simulink model "hydra_tail"  (R2014b)
settings: configuration reference "HardwareConfigLeg" (kept outside this file)
undefined symbols (not defined in the file or in its folder): gcbh, LCD_Status, NXTFcns, R, rmidispblock, Speak, W
libraries: legoev3lib x13, ControllersFcns x5, simulink_extras x4, simulink x3
PreSaveFcn:
  | % Creates new data dictionary based on template.
  | 
  | projRoot = ETRoboconUtilities.getCheckoutRoot;
  | dictName = [bdroot 'Data.sldd'];
  | 
  | source = fullfile(projRoot,'templates','RobotTemplateData.sldd');
  | dest = fullfile(projRoot,'data_dictionaries',dictName);
  | 
  | if ~exist(dest) && ~isequal(bdroot,'RobotTemplate')
  |   copyfile(source,dest);
  |   disp(['Created new dictionary ' dictName ' in the data_dictionaries folder.']);
  |   set_param(bdroot,'DataDictionary', dictName);
  | end
Description:
  | ET Robocon 2014 robot template model.
  | 
  | Author:  Sebastian Castro
settings Model: DataDictionary=hydra_tailData.sldd  ExtModeTrigDuration=2  Creator=mbiesiad  LastModifiedBy=pkaniara

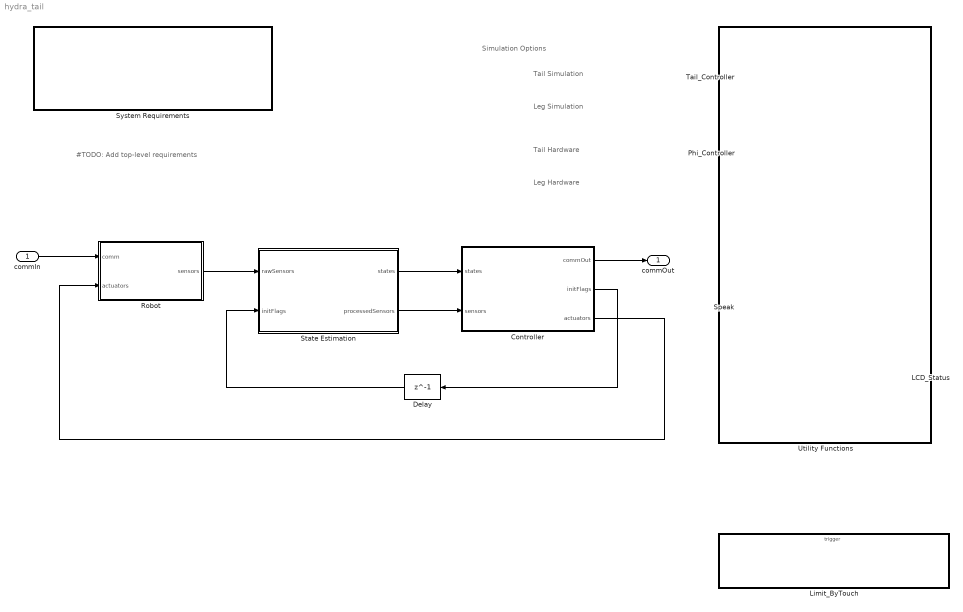
== system hydra_tail ==
  note: #TODO:
      | Add top-level requirements
  note: Simulation Options
  note: Tail Simulation
  note: Tail Hardware
  note: Leg Hardware
  note: Leg Simulation
  commIn : Inport
  Controller : Stateflow chart  TreatAsAtomicUnit=on
  Delay : Delay  DelayLength=1
      settings: AttributesFormatString=Removes algebraic loop
  LCD_Status : Subsystem  AncestorBlock=NXTFcns/LCD_Status  TreatAsAtomicUnit=on
  Limit_ByTouch : Subsystem  TreatAsAtomicUnit=on
  Phi_Controller : ControllersFcns/Phi_Controller
  Robot : Subsystem  Variant=on  VariantControl=Variant1
  Speak : Subsystem  AncestorBlock=NXTFcns/Speak  TreatAsAtomicUnit=on
  State Estimation : Subsystem
  System Requirements : Subsystem  LoadFcn=rmidispblock('load',gcbh)  mask(System Requirements){id=SystemReq, title=System Requirements}
      mask prompts: title "Block Title"
      mask help: Lists the requirements for the current model.
      mask init:
      | id = 'SystemReq';
      | [w,h] = rmidispblock('display',gcbh);
      settings: CopyFcn=rmidispblock('create',gcbh)  DeleteFcn=rmidispblock('delete',gcbh)  ModelCloseFcn=rmidispblock('close',gcbh)  PreSaveFcn=rmidispblock('close',gcbh)  PostSaveFcn=rmidispblock('open',gcbh)  OpenFcn=rmidispblock('open',gcbh)  MoveFcn=rmidispblock('move',gcbh)
      mask Help: helpview(fullfile(docroot,'toolbox','slvnv','slvnv.map'),'systemrequirements')
      mask Display:
      | text(326/2,113-4,rmidispblock('title',gcbh),'horizontalAlignment','center','verticalAlignment','top')
      | text(w/2,h/2,'<No Requirements in System>','horizontalAlignment','center','verticalAlignment','top')
  Tail_Controller : ControllersFcns/Tail_Controller
  Utility Functions : Subsystem
  commOut : Outport
  wires:
  State Estimation/2(processedSensors) -> Controller/2(sensors)
  Robot/1(sensors) -> State Estimation/1(rawSensors)
  Controller/2(initFlags) -> Delay/1
  State Estimation/1(states) -> Controller/1(states)
  Delay/1 -> State Estimation/2(initFlags)
  Controller/3(actuators) -> Robot/2(actuators)
  Controller/1(commOut) -> commOut/1
  commIn/1 -> Robot/1(comm)

== system hydra_tail/Controller/Speak ==
  f : TriggerPort  TriggerType=function-call
      settings: CopyFcn=Stateflow.SLINSF.SimulinkMan.removeBlockPreDeleteFcn  PreDeleteFcn=Stateflow.SLINSF.SimulinkMan.unsafePredeleteFcn
  Constant : Constant  Value=50
  Speaker1 : legoev3lib/Speaker  sinputMode=Volume only  sspeakerFreq=100  sspeakerVolume=50  sspeakerDuration=100
  wires:
  Constant/1 -> Speaker1/1

== system hydra_tail/LCD_Status ==
  StatusLCD : TriggerPort  TriggerType=function-call  IsSimulinkFunction=on  FunctionName=StatusLCD
  Display : legoev3lib/Display  slcdLine=1  slcdFormat=Decimal
  state : ArgIn  OutDataTypeStr=uint16  ArgumentName=state
  wires:
  state/1 -> Display/1

== system hydra_tail/Limit_ByTouch ==
  LimitByTouch : TriggerPort  TriggerType=function-call  IsSimulinkFunction=on  FunctionName=LimitByTouch
  Chart : Stateflow chart  TreatAsAtomicUnit=on
  Compare To Zero : simulink/Logic and Bit Operations/Compare To Zero  relop=>=  OutDataTypeStr=boolean
  Delay : Delay  DelayLength=1
  TouchInput : ArgIn  DisableCoverage=on  ArgumentName=TouchInput
  cmd : ArgOut  DisableCoverage=on  ArgumentName=cmd
  wires:
  TouchInput/1 -> Chart/1(touchInput)
  Chart/1(motorCommand) -> Delay/1, cmd/1
  Delay/1 -> Compare To Zero/1
  Compare To Zero/1 -> Chart/2(direction)

== system hydra_tail/Robot ==
  comm : Inport
  actuators : Inport  Port=2
  EV3 - Legs : Subsystem  VariantControl=HardwareVar2
  EV3 - Tail : Subsystem  VariantControl=HardwareVar1
  Simulation - Legs : Subsystem  VariantControl=SimulationVar2
  Simulation - Tail : Subsystem  VariantControl=SimulationVar1
  sensors : Outport

== system hydra_tail/Speak ==
  Speak : TriggerPort  TriggerType=function-call  IsSimulinkFunction=on  FunctionName=Speak
  Constant : Constant  Value=50
  Speaker1 : legoev3lib/Speaker  sinputMode=Volume only  sspeakerFreq=100  sspeakerVolume=50  sspeakerDuration=100
  wires:
  Constant/1 -> Speaker1/1

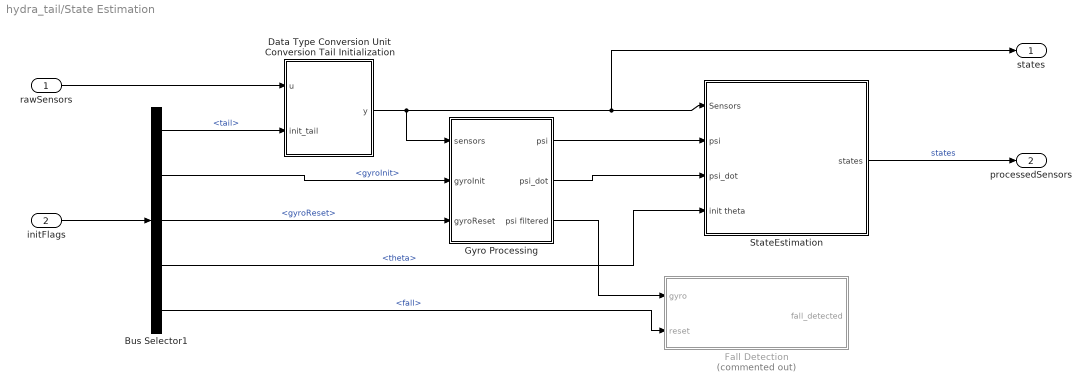
== system hydra_tail/State Estimation ==
  rawSensors : Inport
  initFlags : Inport  Port=2
  Bus Selector1 : BusSelector  OutputSignals=tail,gyroInit,gyroReset,theta,fall
  Data Type Conversion Unit Conversion Tail Initialization : Subsystem
  Fall Detection : Subsystem  Commented=on
  Gyro Processing : Subsystem
  StateEstimation : Subsystem
  states : Outport
  processedSensors : Outport  Port=2
  wires:
  Data Type Conversion Unit Conversion Tail Initialization/1(y) -> Gyro Processing/1(sensors), states/1, StateEstimation/1(Sensors)
  Bus Selector1/3 -> Gyro Processing/3(gyroReset)  "<gyroReset>"
  Bus Selector1/4 -> StateEstimation/4(init theta)  "<theta>"
  Bus Selector1/1 -> Data Type Conversion Unit Conversion Tail Initialization/2(init_tail)  "<tail>"
  Bus Selector1/2 -> Gyro Processing/2(gyroInit)  "<gyroInit>"
  initFlags/1 -> Bus Selector1/1
  StateEstimation/1(states) -> processedSensors/1  "states"
  rawSensors/1 -> Data Type Conversion Unit Conversion Tail Initialization/1(u)
  Gyro Processing/1(psi) -> StateEstimation/2(psi)
  Gyro Processing/2(psi_dot) -> StateEstimation/3(psi_dot)
  Gyro Processing/3(psi filtered) -> Fall Detection/1(gyro)
  Bus Selector1/5 -> Fall Detection/2(reset)  "<fall>"

== system hydra_tail/System Requirements ==
  Subsystem : Subsystem  mask{label=0, index=1}
      mask init:
      | label = rmidispblock('label',index);
      settings: OpenFcn=rmidispblock('openReq',gcbh);
      mask Display: text(0,0,label,'horizontalAlignment','left','verticalAlignment','bottom')

== system hydra_tail/Utility Functions ==

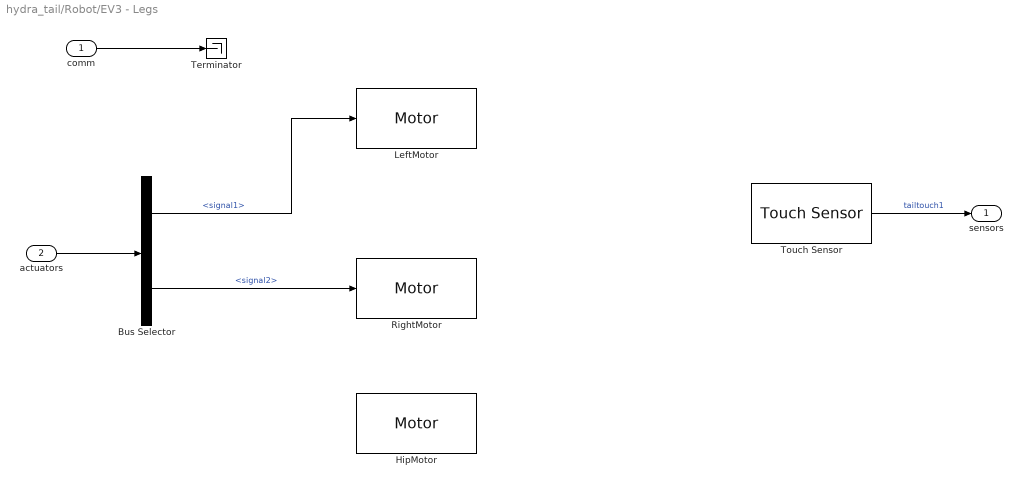
== system hydra_tail/Robot/EV3 - Legs ==
  comm : Inport
  actuators : Inport  Port=2
  Bus Selector : BusSelector  OutputSignals=signal1,signal2
  HipMotor : legoev3lib/Motor  sportNumber=C  sstopAction=Brake
  LeftMotor : legoev3lib/Motor  sportNumber=A  sstopAction=Brake
  RightMotor : legoev3lib/Motor  sportNumber=B  sstopAction=Brake
  Terminator : Terminator
  Touch Sensor : legoev3lib/Touch Sensor  portNumber=1  sampleTime=0.1
  sensors : Outport
  wires:
  comm/1 -> Terminator/1
  Touch Sensor/1 -> sensors/1  "tailtouch1"
  Bus Selector/1 -> LeftMotor/1  "<signal1>"
  actuators/1 -> Bus Selector/1
  Bus Selector/2 -> RightMotor/1  "<signal2>"

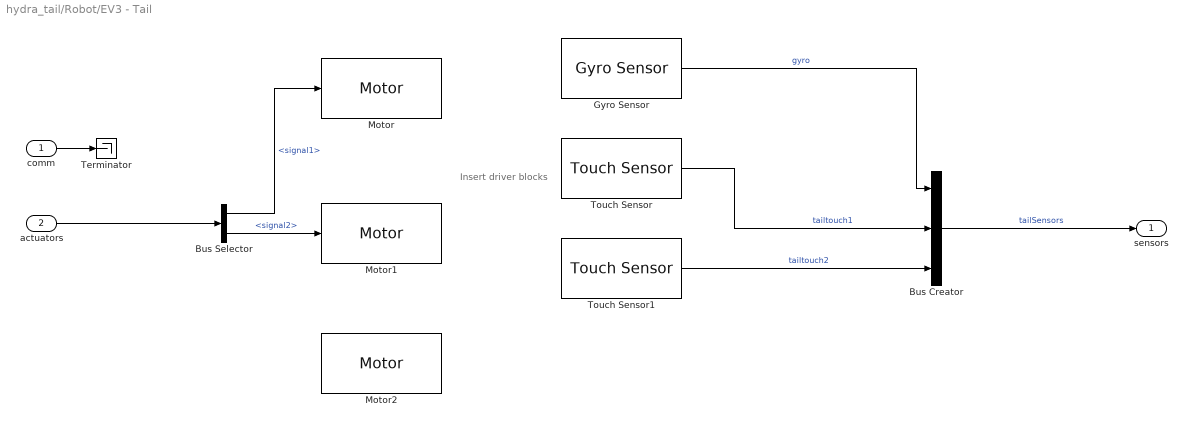
== system hydra_tail/Robot/EV3 - Tail ==
  note: Insert driver blocks
  comm : Inport
  actuators : Inport  Port=2
  Bus Creator : BusCreator  Inputs=3
  Bus Selector : BusSelector  OutputSignals=signal1,signal2
  Gyro Sensor : legoev3lib/Gyro Sensor  portNumber=1  sampleTime=0.1
  Motor : legoev3lib/Motor  sportNumber=A  sstopAction=Brake
  Motor1 : legoev3lib/Motor  sportNumber=B  sstopAction=Brake
  Motor2 : legoev3lib/Motor  sportNumber=C  sstopAction=Brake
  Terminator : Terminator
  Touch Sensor : legoev3lib/Touch Sensor  portNumber=1  sampleTime=0.1
  Touch Sensor1 : legoev3lib/Touch Sensor  portNumber=1  sampleTime=0.1
  sensors : Outport
  wires:
  Bus Creator/1 -> sensors/1  "tailSensors"
  actuators/1 -> Bus Selector/1
  comm/1 -> Terminator/1
  Gyro Sensor/1 -> Bus Creator/1  "gyro"
  Touch Sensor/1 -> Bus Creator/2  "tailtouch1"
  Touch Sensor1/1 -> Bus Creator/3  "tailtouch2"
  Bus Selector/1 -> Motor/1  "<signal1>"
  Bus Selector/2 -> Motor1/1  "<signal2>"

== system hydra_tail/Robot/Simulation - Legs ==
  note: Insert physical model.
      | Talk to the simulation team!
  comm : Inport
  actuators : Inport  Port=2
  Ground : Ground
  Terminator : Terminator
  Terminator1 : Terminator
  sensors : Outport
  wires:
  comm/1 -> Terminator/1
  actuators/1 -> Terminator1/1
  Ground/1 -> sensors/1

== system hydra_tail/Robot/Simulation - Tail ==
  note: Insert physical model.
      | Talk to the simulation team!
  comm : Inport
  actuators : Inport  Port=2
  Ground : Ground
  Terminator : Terminator
  Terminator1 : Terminator
  sensors : Outport
  wires:
  Ground/1 -> sensors/1
  actuators/1 -> Terminator1/1
  comm/1 -> Terminator/1

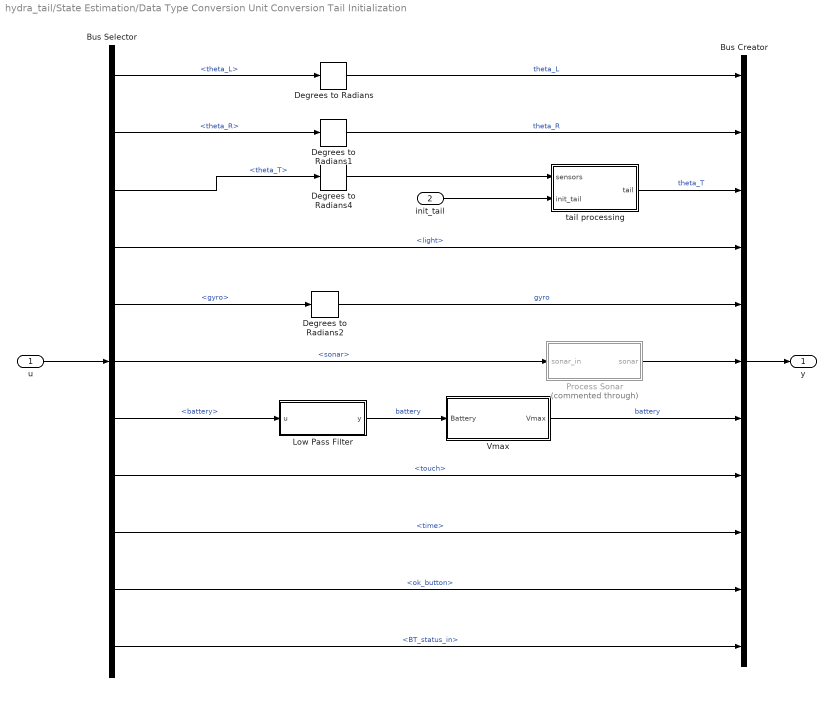
== system hydra_tail/State Estimation/Data Type Conversion Unit Conversion Tail Initialization ==
  u : Inport
  init_tail : Inport  Port=2
  Bus Creator : BusCreator  Inputs=11  OutDataTypeStr=Bus: Sensors_Bus
  Bus Selector : BusSelector  OutputSignals=theta_L,theta_R,theta_T,light,gyro,sonar,battery,touch,time,ok_button,BT_status_in
  Degrees to Radians{,1..2,4} (4 alike) : simulink_extras/Transformations/Degrees to Radians
  Low Pass Filter : Subsystem
  Process Sonar : Subsystem  Commented=through
  Vmax : Subsystem
  tail processing : Subsystem
  y : Outport
  wires:
  Bus Selector/11 -> Bus Creator/11  "<BT_status_in>"
  Process Sonar/1(sonar) -> Bus Creator/6
  Bus Selector/6 -> Process Sonar/1(sonar_in)  "<sonar>"
  Bus Selector/10 -> Bus Creator/10  "<ok_button>"
  init_tail/1 -> tail processing/2(init_tail)
  Bus Selector/9 -> Bus Creator/9  "<time>"
  Bus Selector/8 -> Bus Creator/8  "<touch>"
  tail processing/1(tail) -> Bus Creator/3  "theta_T"
  Degrees to Radians4/1 -> tail processing/1(sensors)
  Vmax/1(Vmax) -> Bus Creator/7  "battery"
  Degrees to Radians2/1 -> Bus Creator/5  "gyro"
  Bus Selector/3 -> Degrees to Radians4/1  "<theta_T>"
  Bus Selector/7 -> Low Pass Filter/1(u)  "<battery>"
  Bus Selector/5 -> Degrees to Radians2/1  "<gyro>"
  Bus Selector/4 -> Bus Creator/4  "<light>"
  Bus Creator/1 -> y/1
  u/1 -> Bus Selector/1
  Degrees to Radians/1 -> Bus Creator/1  "theta_L"
  Bus Selector/2 -> Degrees to Radians1/1  "<theta_R>"
  Bus Selector/1 -> Degrees to Radians/1  "<theta_L>"
  Low Pass Filter/1(y) -> Vmax/1(Battery)  "battery"
  Degrees to Radians1/1 -> Bus Creator/2  "theta_R"

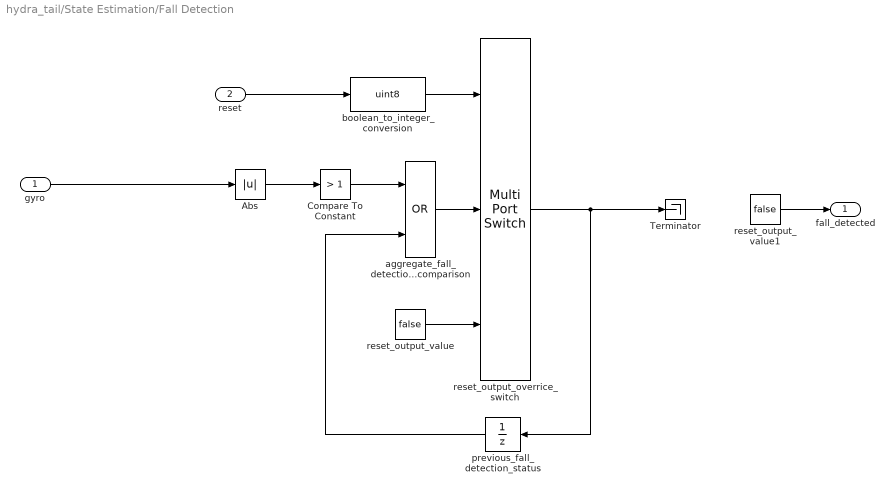
== system hydra_tail/State Estimation/Fall Detection ==
  gyro : Inport
      settings: AttributesFormatString=Output data type: %<OutDataTypeStr>
  reset : Inport  Port=2  OutDataTypeStr=boolean
      settings: AttributesFormatString=Output data type: %<OutDataTypeStr>
  Abs : Abs
  Compare To Constant : simulink/Logic and Bit Operations/Compare To Constant  relop=>  const=1  OutDataTypeStr=boolean
  Terminator : Terminator
  aggregate_fall_detection_comparison : Logic  Operator=OR  OutDataTypeStr=boolean
  boolean_to_integer_conversion : DataTypeConversion  OutDataTypeStr=uint8
      settings: AttributesFormatString=Output data type: %<OutDataTypeStr>
  previous_fall_detection_status : UnitDelay  SampleTime=-1
  reset_output_overrice_switch : MultiPortSwitch  DataPortOrder=Zero-based contiguous  Inputs=2  zeroidx=on  InputSameDT=on
  reset_output_value : Constant  Value=false
  reset_output_value1 : Constant  Value=false  OutDataTypeStr=boolean
  fall_detected : Outport
  wires:
  reset_output_overrice_switch/1 -> Terminator/1, previous_fall_detection_status/1
  reset_output_value/1 -> reset_output_overrice_switch/3
  aggregate_fall_detection_comparison/1 -> reset_output_overrice_switch/2
  boolean_to_integer_conversion/1 -> reset_output_overrice_switch/1
  reset/1 -> boolean_to_integer_conversion/1
  previous_fall_detection_status/1 -> aggregate_fall_detection_comparison/2
  Abs/1 -> Compare To Constant/1
  gyro/1 -> Abs/1
  Compare To Constant/1 -> aggregate_fall_detection_comparison/1
  reset_output_value1/1 -> fall_detected/1

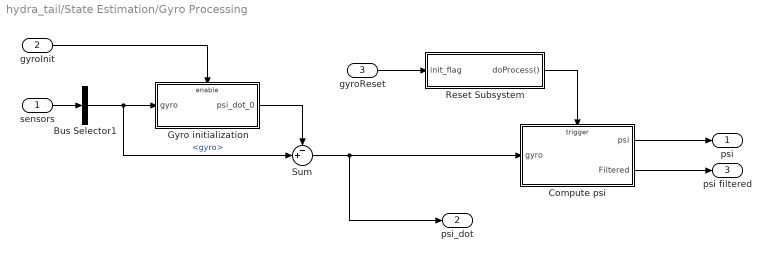
== system hydra_tail/State Estimation/Gyro Processing ==
  sensors : Inport
  gyroInit : Inport  Port=2
  gyroReset : Inport  Port=3
  Bus Selector1 : BusSelector  OutputSignals=gyro
  Compute psi : Subsystem
  Gyro initialization : Subsystem  TreatAsAtomicUnit=on
  Reset Subsystem : Stateflow chart  TreatAsAtomicUnit=on
  Sum : Sum  Inputs=-+|
  psi : Outport
  psi_dot : Outport  Port=2
  psi filtered : Outport  Port=3
  wires:
  Compute psi/2(Filtered) -> psi filtered/1
  Reset Subsystem/1(doProcess()) -> Compute psi/Trigger
  gyroReset/1 -> Reset Subsystem/1(init_flag)
  Bus Selector1/1 -> Sum/2, Gyro initialization/1(gyro)  "<gyro>"
  Gyro initialization/1(psi_dot_0) -> Sum/1
  Sum/1 -> psi_dot/1, Compute psi/1(gyro)
  Compute psi/1(psi) -> psi/1
  sensors/1 -> Bus Selector1/1
  gyroInit/1 -> Gyro initialization/Enable

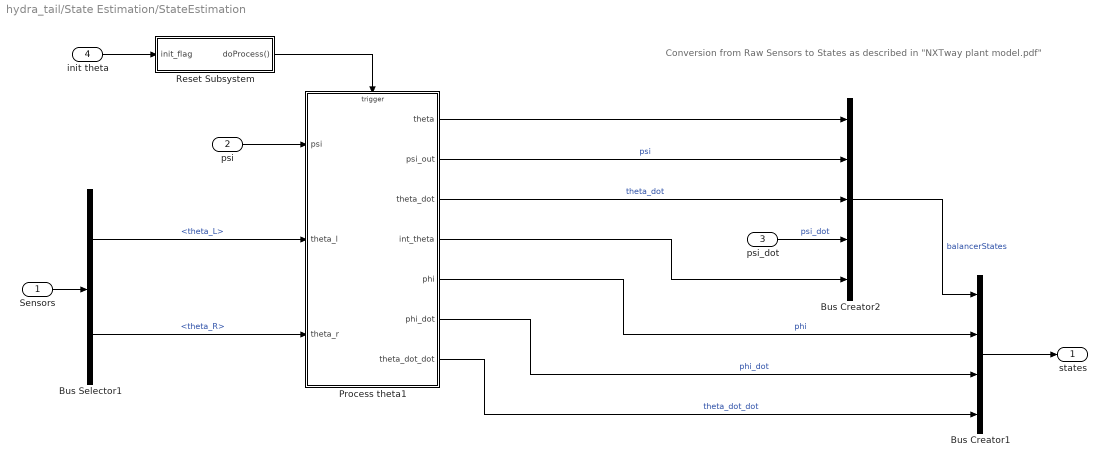
== system hydra_tail/State Estimation/StateEstimation ==
  note: Conversion from Raw Sensors to States as described in "NXTway plant model.pdf"
  Sensors : Inport
  psi : Inport  Port=2
  psi_dot : Inport  Port=3
  init theta : Inport  Port=4
  Bus Creator1 : BusCreator  OutDataTypeStr=Bus: States_Bus
  Bus Creator2 : BusCreator  Inputs=5  OutDataTypeStr=Bus: Balancer_States_Bus
  Bus Selector1 : BusSelector  OutputSignals=theta_L,theta_R
  Process theta1 : Subsystem
  Reset Subsystem : Stateflow chart  TreatAsAtomicUnit=on
  states : Outport  OutputWhenDisabled=reset  InitialOutput=0
  wires:
  Process theta1/2(psi_out) -> Bus Creator2/2  "psi"
  Reset Subsystem/1(doProcess()) -> Process theta1/Trigger
  Bus Selector1/2 -> Process theta1/3(theta_r)  "<theta_R>"
  Bus Selector1/1 -> Process theta1/2(theta_l)  "<theta_L>"
  init theta/1 -> Reset Subsystem/1(init_flag)
  Process theta1/1(theta) -> Bus Creator2/1
  Process theta1/3(theta_dot) -> Bus Creator2/3  "theta_dot"
  Process theta1/4(int_theta) -> Bus Creator2/5
  psi_dot/1 -> Bus Creator2/4  "psi_dot"
  Process theta1/6(phi_dot) -> Bus Creator1/3  "phi_dot"
  Bus Creator2/1 -> Bus Creator1/1  "balancerStates"
  Process theta1/5(phi) -> Bus Creator1/2  "phi"
  Sensors/1 -> Bus Selector1/1
  psi/1 -> Process theta1/1(psi)
  Bus Creator1/1 -> states/1
  Process theta1/7(theta_dot_dot) -> Bus Creator1/4  "theta_dot_dot"

== system hydra_tail/System Requirements/Subsystem ==

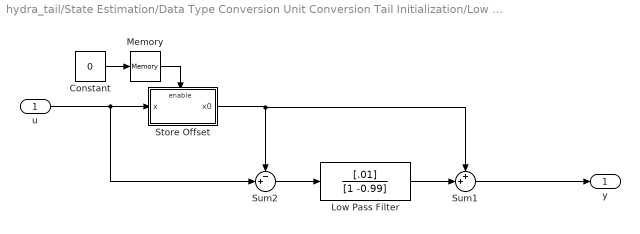
== system hydra_tail/State Estimation/Data Type Conversion Unit Conversion Tail Initialization/Low Pass Filter ==
  u : Inport
  Constant : Constant  Value=0  OutDataTypeStr=boolean
  Low Pass Filter : DiscreteFilter  Numerator=[.01]  Denominator=[1 -0.99]
  Memory : Memory  X0=1  InheritSampleTime=on
  Store Offset : Subsystem  TreatAsAtomicUnit=on
  Sum1 : Sum  Inputs=++|
  Sum2 : Sum  Inputs=-+|
  y : Outport
  wires:
  Store Offset/1(x0) -> Sum1/1, Sum2/1
  u/1 -> Store Offset/1(x), Sum2/2
  Constant/1 -> Memory/1
  Memory/1 -> Store Offset/Enable
  Sum2/1 -> Low Pass Filter/1
  Sum1/1 -> y/1
  Low Pass Filter/1 -> Sum1/2

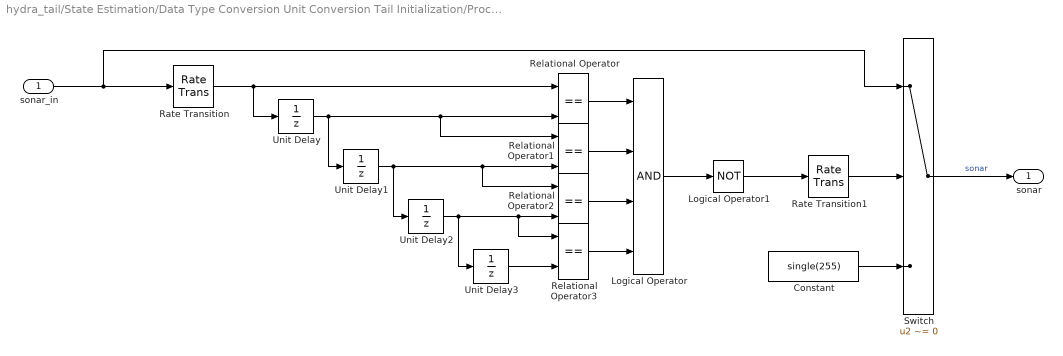
== system hydra_tail/State Estimation/Data Type Conversion Unit Conversion Tail Initialization/Process Sonar ==
  sonar_in : Inport
  Constant : Constant  Value=single(255)
  Logical Operator : Logic  Inputs=4  AllPortsSameDT=off  OutDataTypeStr=boolean
  Logical Operator1 : Logic  Operator=NOT  AllPortsSameDT=off  OutDataTypeStr=boolean
  Rate Transition : RateTransition  OutPortSampleTime=0.02
  Rate Transition1 : RateTransition  OutPortSampleTime=0.004
  Relational Operator{,1..3} (4 alike) : RelationalOperator  Operator===  OutDataTypeStr=boolean
  Switch : Switch  Criteria=u2 ~= 0
  Unit Delay{,1..3} (4 alike) : UnitDelay  SampleTime=-1
  sonar : Outport
  wires:
  Switch/1 -> sonar/1  "sonar"
  Constant/1 -> Switch/3
  Rate Transition1/1 -> Switch/2
  Logical Operator1/1 -> Rate Transition1/1
  Logical Operator/1 -> Logical Operator1/1
  Relational Operator2/1 -> Logical Operator/3
  Relational Operator1/1 -> Logical Operator/2
  Relational Operator3/1 -> Logical Operator/4
  Relational Operator/1 -> Logical Operator/1
  Unit Delay3/1 -> Relational Operator3/2
  Unit Delay2/1 -> Unit Delay3/1, Relational Operator2/2, Relational Operator3/1
  Unit Delay1/1 -> Unit Delay2/1, Relational Operator1/2, Relational Operator2/1
  Unit Delay/1 -> Unit Delay1/1, Relational Operator/2, Relational Operator1/1
  Rate Transition/1 -> Unit Delay/1, Relational Operator/1
  sonar_in/1 -> Rate Transition/1, Switch/1

== system hydra_tail/State Estimation/Data Type Conversion Unit Conversion Tail Initialization/Vmax ==
  Battery : Inport
  Constant : Constant  Value=0.625  OutDataTypeStr=single
  Gain1 : Gain  Gain=0.001089
  Sum : Sum  Inputs=|+-
  Vmax : Outport
  wires:
  Battery/1 -> Gain1/1
  Gain1/1 -> Sum/1
  Constant/1 -> Sum/2
  Sum/1 -> Vmax/1

== system hydra_tail/State Estimation/Data Type Conversion Unit Conversion Tail Initialization/tail processing ==
  sensors : Inport
  init_tail : Inport  Port=2
  Sum : Sum  Inputs=-+|
  tail initialization : Subsystem  TreatAsAtomicUnit=on
  tail : Outport  OutputWhenDisabled=reset  InitialOutput=0
  wires:
  Sum/1 -> tail/1  "theta_T"
  sensors/1 -> Sum/2, tail initialization/1(tail)
  tail initialization/1(tail_0) -> Sum/1
  init_tail/1 -> tail initialization/Trigger

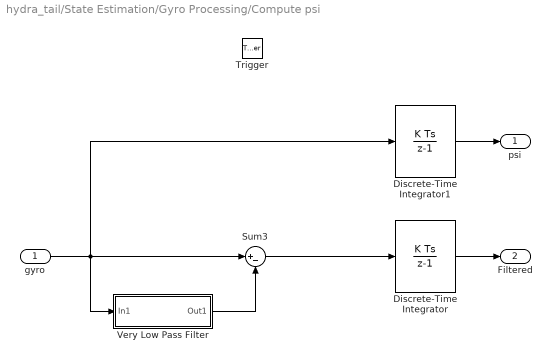
== system hydra_tail/State Estimation/Gyro Processing/Compute psi ==
  gyro : Inport
  Trigger : TriggerPort  TriggerType=function-call  StatesWhenEnabling=reset  PortDimensions=1
  Discrete-Time Integrator : DiscreteIntegrator  SampleTime=-1
  Discrete-Time Integrator1 : DiscreteIntegrator  SampleTime=-1
  Sum3 : Sum  Inputs=|+-
  Very Low Pass Filter : Subsystem
  psi : Outport  InitialOutput=0
  Filtered : Outport  Port=2  InitialOutput=0
  wires:
  Discrete-Time Integrator/1 -> Filtered/1
  Discrete-Time Integrator1/1 -> psi/1
  Sum3/1 -> Discrete-Time Integrator/1
  Very Low Pass Filter/1(Out1) -> Sum3/2
  gyro/1 -> Very Low Pass Filter/1(In1), Sum3/1, Discrete-Time Integrator1/1

== system hydra_tail/State Estimation/Gyro Processing/Gyro initialization ==
  gyro : Inport
  Enable : EnablePort  StatesWhenEnabling=reset
  Low Pass Filter : DiscreteFilter  Numerator=[.01]  Denominator=[1 -0.99]
  psi_dot_0 : Outport  InitialOutput=0
  wires:
  Low Pass Filter/1 -> psi_dot_0/1
  gyro/1 -> Low Pass Filter/1

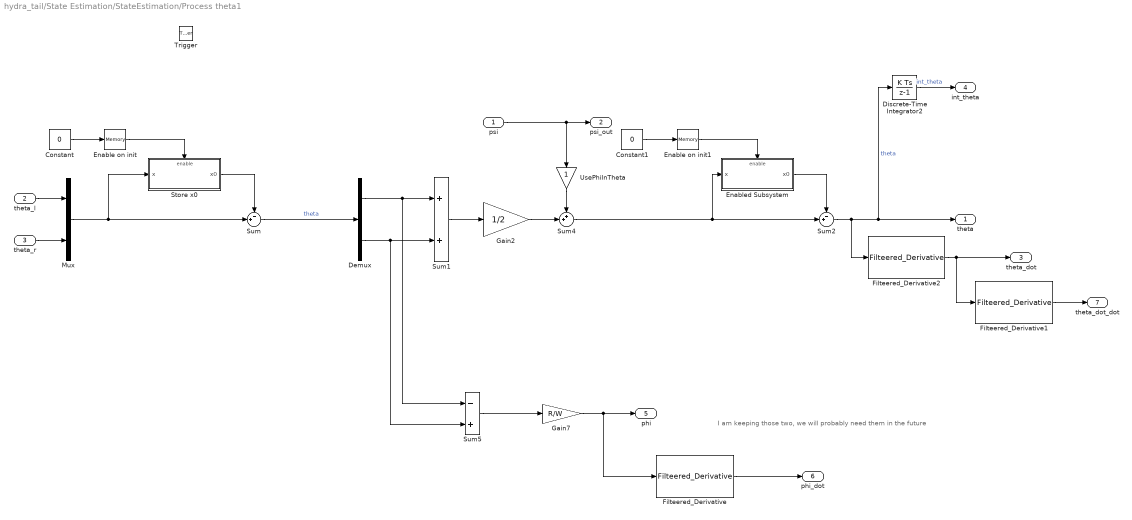
== system hydra_tail/State Estimation/StateEstimation/Process theta1 ==
  note: I am keeping those two, we will probably need them in the future
  psi : Inport
  theta_l : Inport  Port=2
  theta_r : Inport  Port=3
  Trigger : TriggerPort  TriggerType=function-call  StatesWhenEnabling=reset  PortDimensions=1
  Constant : Constant  Value=0  OutDataTypeStr=boolean
  Constant1 : Constant  Value=0  OutDataTypeStr=boolean
  Demux : Demux  Outputs=2
  Discrete-Time Integrator2 : DiscreteIntegrator  SampleTime=-1
  Enable on init : Memory  X0=1  InheritSampleTime=on
  Enable on init1 : Memory  X0=1  InheritSampleTime=on
  Enabled Subsystem : Subsystem  TreatAsAtomicUnit=on
  Filteered_Derivative : ControllersFcns/Filteered_Derivative
  Filteered_Derivative1 : ControllersFcns/Filteered_Derivative
  Filteered_Derivative2 : ControllersFcns/Filteered_Derivative
  Gain2 : Gain  Gain=1/2
  Gain7 : Gain  Gain=R/W
  Mux : Mux  Inputs=2
  Store x0 : Subsystem  TreatAsAtomicUnit=on
  Sum : Sum  Inputs=-+|
  Sum1 : Sum
  Sum2 : Sum  Inputs=-+|
  Sum4 : Sum  Inputs=++|
  Sum5 : Sum  Inputs=-+
  UsePhiInTheta : Gain
  theta : Outport  InitialOutput=0
  psi_out : Outport  Port=2  InitialOutput=0
  theta_dot : Outport  Port=3  OutputWhenDisabled=reset  InitialOutput=0
  int_theta : Outport  Port=4  InitialOutput=0
  phi : Outport  Port=5  OutputWhenDisabled=reset  InitialOutput=0
  phi_dot : Outport  Port=6  OutputWhenDisabled=reset  InitialOutput=0
  theta_dot_dot : Outport  Port=7  OutputWhenDisabled=reset  InitialOutput=0
  wires:
  Gain7/1 -> Filteered_Derivative/1, phi/1
  Sum5/1 -> Gain7/1
  Sum2/1 -> Filteered_Derivative2/1, theta/1, Discrete-Time Integrator2/1  "theta"
  Enabled Subsystem/1(x0) -> Sum2/1
  Constant1/1 -> Enable on init1/1
  Enable on init1/1 -> Enabled Subsystem/Enable
  Sum4/1 -> Sum2/2, Enabled Subsystem/1(x)
  Discrete-Time Integrator2/1 -> int_theta/1  "int_theta"
  psi/1 -> UsePhiInTheta/1, psi_out/1
  UsePhiInTheta/1 -> Sum4/1
  Sum1/1 -> Gain2/1
  Gain2/1 -> Sum4/2
  Demux/2 -> Sum1/2, Sum5/2
  Demux/1 -> Sum1/1, Sum5/1
  theta_r/1 -> Mux/2
  theta_l/1 -> Mux/1
  Mux/1 -> Sum/2, Store x0/1(x)
  Sum/1 -> Demux/1  "theta"
  Store x0/1(x0) -> Sum/1
  Constant/1 -> Enable on init/1
  Enable on init/1 -> Store x0/Enable
  Filteered_Derivative/1 -> phi_dot/1
  Filteered_Derivative2/1 -> Filteered_Derivative1/1, theta_dot/1
  Filteered_Derivative1/1 -> theta_dot_dot/1

== system hydra_tail/State Estimation/Data Type Conversion Unit Conversion Tail Initialization/Low Pass Filter/Store Offset ==
  x : Inport
  Enable : EnablePort
  x0 : Outport  InitialOutput=0
  wires:
  x/1 -> x0/1

== system hydra_tail/State Estimation/Data Type Conversion Unit Conversion Tail Initialization/tail processing/tail initialization ==
  tail : Inport
  Trigger : TriggerPort  PortDimensions=1
  tail_0 : Outport  InitialOutput=0
  wires:
  tail/1 -> tail_0/1

== system hydra_tail/State Estimation/Gyro Processing/Compute psi/Very Low Pass Filter ==
  In1 : Inport
  Gain2 : Gain  Gain=0.004
  Gain3 : Gain  Gain=0.996
  Sum2 : Sum  Inputs=|++
  Unit Delay External IC : simulink/Additional Math & Discrete/Additional Discrete/Unit Delay External IC  tsamp=-1
  Out1 : Outport
  wires:
  Gain3/1 -> Sum2/2
  Sum2/1 -> Out1/1, Unit Delay External IC/1
  Gain2/1 -> Sum2/1
  Unit Delay External IC/1 -> Gain3/1
  In1/1 -> Gain2/1, Unit Delay External IC/2

== system hydra_tail/State Estimation/StateEstimation/Process theta1/Enabled Subsystem ==
  x : Inport
  Enable : EnablePort
  x0 : Outport  InitialOutput=0
  wires:
  x/1 -> x0/1

== system hydra_tail/State Estimation/StateEstimation/Process theta1/Store x0 ==
  x : Inport
  Enable : EnablePort
  x0 : Outport  InitialOutput=0
  wires:
  x/1 -> x0/1

== stateflow chart hydra_tail/State Estimation/Gyro Processing/Reset Subsystem ==
  state CheckForReset
    bind: doProcess;
    entry: doProcess;
    during: doProcess;
  (default) -> CheckForReset
  CheckForReset -> CheckForReset : [init_flag == 1]
  data: init_flag input
  events: doProcess output FUNCTION_CALL_EVENT

== stateflow chart hydra_tail/State Estimation/StateEstimation/Reset Subsystem ==
  state CheckForReset
    bind: doProcess;
    entry: doProcess;
    during: doProcess;
  (default) -> CheckForReset
  CheckForReset -> CheckForReset : [init_flag == 1]
  data: init_flag input
  events: doProcess output FUNCTION_CALL_EVENT

== stateflow chart hydra_tail/Limit_ByTouch/Chart ==
  state Clockwise
    en,du:
    motorCommand = 20;
  state AntiClockwise
    en,du:
    motorCommand = -20;
  AntiClockwise -> Clockwise : [direction==0 && touchInput ==1]
  Clockwise -> AntiClockwise : [direction==1 && touchInput ==1]
  data: touchInput input; motorCommand output; direction input

== stateflow chart hydra_tail/Controller ==
  note: #TODO
      | Add requirements to Stateflow objects
      | by right-clicking and selecting the
      | Requirements Traceability option.
  state Tail Balance
    % Add control logic here.
  state Speak [function]
  (default) -> Tail Balance
  data: commOut output single size=1; states input Bus: States_Bus size=1; sensors input Bus: Sensors_Bus size=1; initFlags output Bus: Init_Bus size=1; actuators output Bus: Actuators_bus size=1
